simulink model "EEL_5661_F22_bicycle_092222"  (R2019a)
settings: Solver=VariableStepAuto  StartTime=0.0  StopTime=10.0  RelTol=1e-3
libraries: simulink x1
settings Model: Creator=rothz  LastModifiedBy=rothz

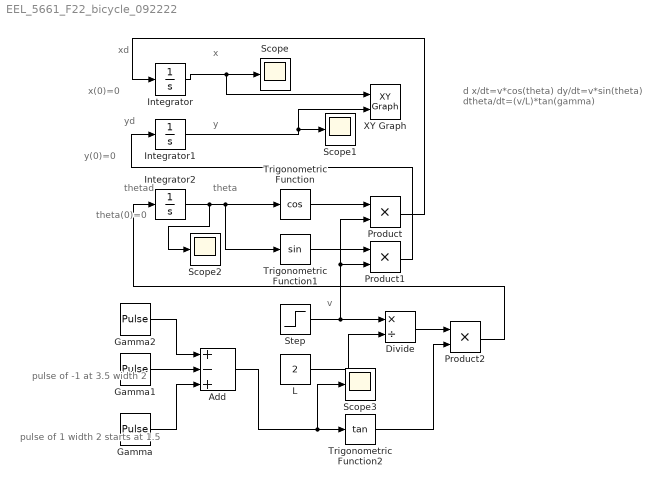
== system EEL_5661_F22_bicycle_092222 ==
  note: pulse of -1 at 3.5
      | width 2
  note: pulse of 1 width 2
      | starts at 1.5
  note: theta(0)=0
  note: y(0)=0
  note: x(0)=0
  note: v
  note: thetad
  note: yd
  note: xd
  note: theta
  note: y
  note: x
  note: d x/dt=v*cos(theta)
      | dy/dt=v*sin(theta)
      | dtheta/dt=(v/L)*tan(gamma)
  Add : Sum  Inputs=+-+
  Divide : Product  Inputs=*/
  Gamma : DiscretePulseGenerator  PulseType=Time based  Period=20  PulseWidth=10  PhaseDelay=1.5
  Gamma1 : DiscretePulseGenerator  PulseType=Time based  Period=20  PulseWidth=10  PhaseDelay=3.5
  Gamma2 : DiscretePulseGenerator  PulseType=Time based  Period=20  PulseWidth=10  PhaseDelay=20
  Integrator : Integrator
  Integrator1 : Integrator
  Integrator2 : Integrator
  L : Constant  Value=2
  Product : Product
  Product1 : Product
  Product2 : Product
  Scope{,1..3} (4 alike) : Scope
  Step : Step  SampleTime=0
  Trigonometric Function : Trigonometry  Operator=cos
  Trigonometric Function1 : Trigonometry
  Trigonometric Function2 : Trigonometry  Operator=tan
  XY Graph : simulink/Sinks/XY Graph  xmin=-1  xmax=10  ymin=-1  ymax=5  st=-1
  wires:
  Integrator2/1 -> Scope2/1, Trigonometric Function1/1, Trigonometric Function/1
  Trigonometric Function/1 -> Product/1
  Step/1 -> Divide/1, Product/2, Product1/2
  Trigonometric Function1/1 -> Product1/1
  Product/1 -> Integrator/1
  Product1/1 -> Integrator1/1
  Integrator/1 -> XY Graph/1, Scope/1
  Integrator1/1 -> XY Graph/2, Scope1/1
  L/1 -> Divide/2
  Divide/1 -> Product2/1
  Trigonometric Function2/1 -> Product2/2
  Product2/1 -> Integrator2/1
  Gamma/1 -> Add/3
  Gamma1/1 -> Add/2
  Gamma2/1 -> Add/1
  Add/1 -> Scope3/1, Trigonometric Function2/1
